simulink model "Test_StateSpace"  (R2013b)
settings: Solver=ode45  StartTime=0.0  StopTime=200  RelTol=1e-3
libraries: dspadpt3 x1, simulink_extras x1, simulink x1
settings Model: Creator=ANKITA003  LastModifiedBy=ANKITA003

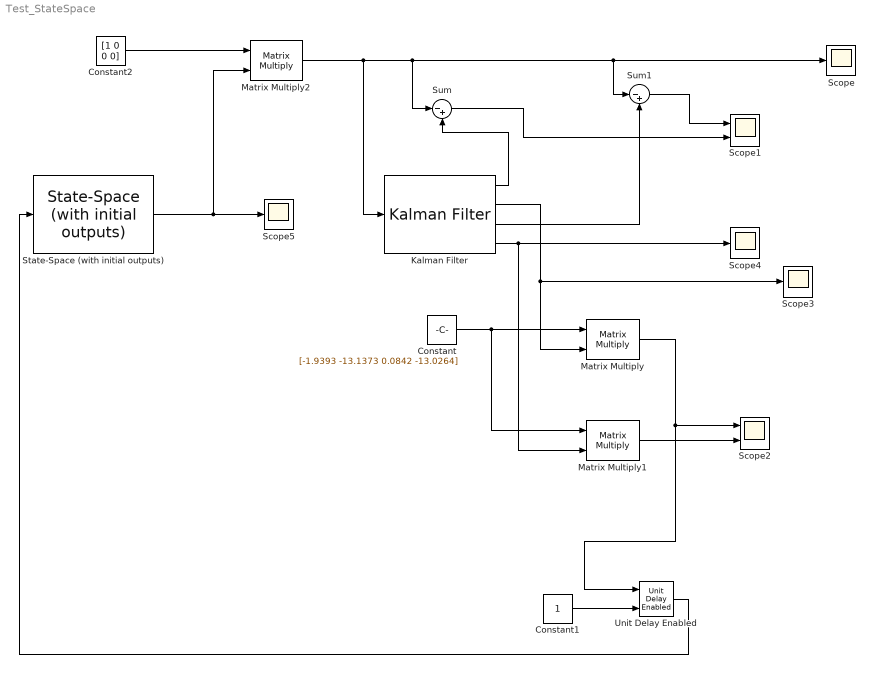
== system Test_StateSpace ==
  Constant : Constant  Value=[-1.9393 -13.1373 0.0842 -13.0264]  VectorParams1D=off  SampleTime=1
  Constant1 : Constant
  Constant2 : Constant  Value=[1 0 0 0]  VectorParams1D=off  SampleTime=1
  Kalman Filter : dspadpt3/Kalman Filter  num_targets=1  sourceEnable=Always  isReset=on  X=zeros([4, 1])  P=10*eye(4)  A=[1 1 0 0;0 1 0 0;0 0 1 1;0 0 0 1]  sourceMeasure=Specify via Dialog  H=[1 0 0 0]  Q=0.05*eye(4)  R=1.8  isOutputEstMeasure=on  isOutputEstState=on  isOutputEstError=off  isOutputPrdMeasure=on  isOutputPrdState=on  isOutputPrdError=off
  Matrix Multiply : Product  Multiplication=Matrix(*)
  Matrix Multiply1 : Product  Multiplication=Matrix(*)
  Matrix Multiply2 : Product  Multiplication=Matrix(*)
  Scope{,3..5} (4 alike) : Scope
      Scope3 settings: SaveName=ScopeData3
      Scope4 settings: SaveName=ScopeData4
      Scope5 settings: SaveName=ScopeData5
  Scope1 : Scope  NumInputPorts=2
      settings: YMin=-5~-5  YMax=5~5
  Scope2 : Scope  NumInputPorts=2
      settings: YMin=-5~-5  YMax=5~5  SaveName=ScopeData2
  State-Space (with initial outputs) : simulink_extras/Additional Linear/State-Space (with initial outputs)  A=[0 1.0000 0 0;0 -1.6500 0.5000 1.0000;0 0 0 1.0000;0 1.5000 -0.5000 -1.0000]  B=[0;0.1100;0;-0.1000]  C=[1 0 0 0;0 1 0 0;0 0 1 0;0 0 0 1]  D=[0; 0; 0; 0]  U0=-1  Y0=0
  Sum : Sum  Inputs=|-+  SampleTime=1
  Sum1 : Sum  Inputs=|-+  SampleTime=1
  Unit Delay Enabled : simulink/Additional Math & Discrete/Additional Discrete/Unit Delay Enabled  vinit=1  tsamp=1
  wires:
  State-Space (with initial outputs)/1 -> Scope5/1, Matrix Multiply2/2
  Matrix Multiply1/1 -> Scope2/2
  Kalman Filter/1 -> Sum/2
  Kalman Filter/3 -> Sum1/2
  Sum/1 -> Scope1/2
  Sum1/1 -> Scope1/1
  Constant/1 -> Matrix Multiply1/1, Matrix Multiply/1
  Kalman Filter/2 -> Scope3/1, Matrix Multiply/2
  Kalman Filter/4 -> Scope4/1, Matrix Multiply1/2
  Matrix Multiply/1 -> Unit Delay Enabled/1, Scope2/1
  Unit Delay Enabled/1 -> State-Space (with initial outputs)/1
  Constant1/1 -> Unit Delay Enabled/2
  Constant2/1 -> Matrix Multiply2/1
  Matrix Multiply2/1 -> Kalman Filter/1, Sum/1, Sum1/1, Scope/1
